simulink model "vision_processing"  (Simulink 7.7)
settings: Solver=FixedStepDiscrete  StartTime=0.0  StopTime=inf  FixedStep=0.05  RelTol=1e-3
undefined symbols (not defined in the file): darwinop_communication_setup
libraries: simulink x16, lib_darwinop x1
settings Model: Creator=florent  LastModifiedBy=eleve
settings DataIOCC: SignalLoggingSaveFormat=Dataset
settings OptimizationCC: ExpressionDepthLimit=128  OptimizeModelRefInitCode=on  LifeSpan=1
settings DebuggingCC: FcnCallInpInsideContextMsg=Enable All
settings HardwareCC: ProdEndianess=LittleEndian  ProdHWDeviceType=Generic->32-bit Embedded Processor
settings RTWCC: SystemTargetFile=darwinoplib.tlc  GenCodeOnly=on  TemplateMakefile=darwinoplib.tmf  Description=DarwinOP code generator  ProcessScript=darwinoplib_make_rtw_hook  TargetLang=C++
settings CodeAppCC: IgnoreCustomStorageClasses=off  CustomSymbolStrType=$N$R$M_T
settings STFCustomTargetCC: CombineOutputUpdateFcns=on  ERTCustomFileBanners=on  SupportContinuousTime=off  SupportNonInlinedSFcns=off  SystemTargetFile=darwinoplib.tlc
settings ERTTargetCC: MultiwordLength=2048  ParMdlRefBuildCompliant=off  CompOptLevelCompliant=off  ERTFirstTimeCompliant=off  ModelStepFunctionPrototypeControlCompliant=off  CPPClassGenCompliant=off  ExtModeMexArgs='192.168.123.1' 1 17725  InlinedParameterPlacement=NonHierarchical  ERTCustomFileTemplate=darwinoplib_main.tlc  ConvertIfToSwitch=off  SuppressUnreachableDefaultCases=off
settings CustomProperty: DataType=string  Value=192.168.123.1

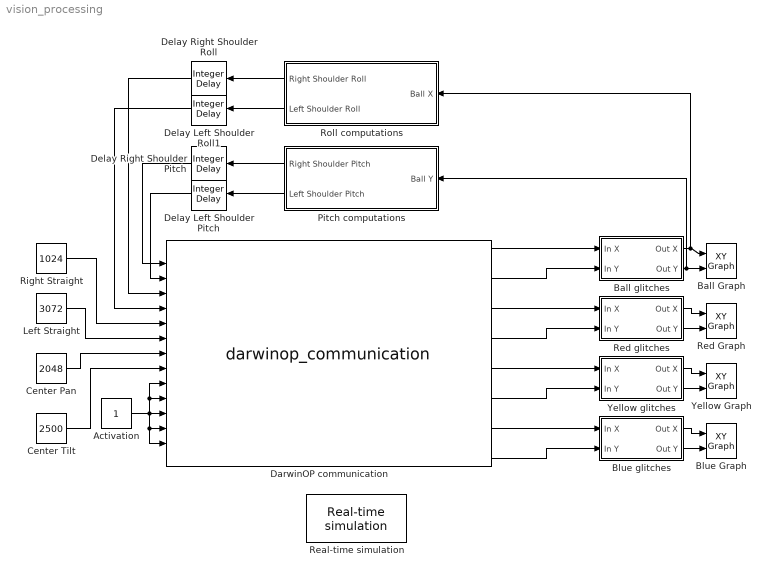
== system vision_processing ==
  Activation : Constant
  Ball Graph : simulink/Sinks/XY Graph  xmin=0  xmax=320  ymin=0  ymax=240  st=-1
  Ball glitches : Subsystem
  Blue Graph : simulink/Sinks/XY Graph  xmin=0  xmax=320  ymin=0  ymax=240  st=-1
  Blue glitches : Subsystem
  Center Pan : Constant  Value=2048
  Center Tilt : Constant  Value=2500
  DarwinOP communication : M-S-Function  StartFcn=darwinop_communication_setup('StartFcn');  StopFcn=darwinop_communication_setup('StopFcn');  FunctionName=darwinop_communication  Parameters=IP,Port,Protocol,Timeout,Frame,ReadIndex,WriteIndex  mask{IP=192.168.123.1, Port=1234, Protocol=tcp, Timeout=0.05, Frame=[ 3 1 30 2 0 0 3 2 30 2 0 0 3 3 30 2 0 0 3 4 30 2 0 0 3 5 30 2 0 0 3 6 30 2 0 0 3 19 30 2 0 0 3 20 30 2 0 0 17 1 30 4 17 1 50 4 17 1 70 4 17 1 90 4 18 1 1 5 0 0 0 0 0], ReadIndex=[ 1 2;3 2;5 2;7 2;9 2;11 2;13 2;15 2], WriteIndex=[ 5 2;11 2;17 2;23 2;29 2;35 2;41 2;47 2;69 1;70 1;71 1;72 1;73 1]}
      settings: DeleteFcn=darwinop_communication_setup('DeleteFcn');  ModelCloseFcn=darwinop_communication_setup('ModelCloseFcn');  NameChangeFcn=darwinop_communication_setup('NameChangeFcn');  OpenFcn=darwinop_communication_setup('OpenFcn');
      mask StyleString: edit,edit,popup(tcp|udp),edit,edit,edit,edit
      mask Display:
      | image(imread('darwin-blk.jpg'))
      | 
      | port_label('output',1,'Vision(1)/Ball X')
      | port_label('output',2,'Vision(1)/Ball Y')
      | port_label('output',3,'Vision(1)/Red X')
      | port_label('output',4,'Vision(1)/Red Y')
      | port_label('output',5,'Vision(1)/Yellow X')
      | port_label('output',6,'Vision(1)/Yellow Y')
      | port_label('output',7,'Vision(1)/Blue X')
      | port_label('output',8,'Vision(1)/Blue Y')
      | 
      | port_label('input',1,'Right Shoulder Pitch(1)/Goal Position')
      | port_label('input',2,'Left Shoulder Pitch(2)/Goal Position')
      | port_label('input',3,'Right Shoulder Roll(3)/Goal Position')
      | port_label('input',4,'Left Shoulder Roll(4)/Goal Position')
      | port_label('input',5,'Right Elbow(5)/Goal Position')
      | port_label('input',6,'Left Elbow(6)/Goal Position')
      | port_label('input',7,'Head Pan(19)/Goal Position')
      | port_label('input',8,'Head Tilt(20)/Goal Position')
      | port_label('input',9,'Vision(1)/Enable')
      | port_label('input',10,'Vision(1)/Ball enable')
      | port_label('input',11,'Vision(1)/Red enable')
      | port_label('input',12,'Vision(1)/Yellow enable')
      | port_label('input',13,'Vision(1)/Blue enable')
  Delay Left Shoulder Pitch : simulink/Discrete/Integer Delay  NumDelays=1  vinit=2048  samptime=-1
  Delay Left Shoulder Roll1 : simulink/Discrete/Integer Delay  NumDelays=1  vinit=2048  samptime=-1
  Delay Right Shoulder Pitch : simulink/Discrete/Integer Delay  NumDelays=1  vinit=2048  samptime=-1
  Delay Right Shoulder Roll : simulink/Discrete/Integer Delay  NumDelays=1  vinit=2048  samptime=-1
  Left Straight : Constant  Value=3072
  Pitch computations : Subsystem
  Real-time simulation : lib_darwinop/Real-time simulation  TimeScalingFactor=1
  Red Graph : simulink/Sinks/XY Graph  xmin=0  xmax=320  ymin=0  ymax=240  st=-1
  Red glitches : Subsystem
  Right Straight : Constant  Value=1024
  Roll computations : Subsystem
  Yellow Graph : simulink/Sinks/XY Graph  xmin=0  xmax=320  ymin=0  ymax=240  st=-1
  Yellow glitches : Subsystem
  wires:
  DarwinOP communication/1 -> Ball glitches/1(In X)
  Ball glitches/1(Out X) -> Roll computations/1(Ball X), Ball Graph/1
  DarwinOP communication/2 -> Ball glitches/2(In Y)
  Ball glitches/2(Out Y) -> Pitch computations/1(Ball Y), Ball Graph/2
  DarwinOP communication/3 -> Red glitches/1(In X)
  Red glitches/1(Out X) -> Red Graph/1
  DarwinOP communication/4 -> Red glitches/2(In Y)
  Red glitches/2(Out Y) -> Red Graph/2
  DarwinOP communication/5 -> Yellow glitches/1(In X)
  Yellow glitches/1(Out X) -> Yellow Graph/1
  DarwinOP communication/6 -> Yellow glitches/2(In Y)
  Yellow glitches/2(Out Y) -> Yellow Graph/2
  DarwinOP communication/7 -> Blue glitches/1(In X)
  Blue glitches/1(Out X) -> Blue Graph/1
  DarwinOP communication/8 -> Blue glitches/2(In Y)
  Blue glitches/2(Out Y) -> Blue Graph/2
  Activation/1 -> DarwinOP communication/10, DarwinOP communication/9, DarwinOP communication/11, DarwinOP communication/12, DarwinOP communication/13
  Center Pan/1 -> DarwinOP communication/7
  Right Straight/1 -> DarwinOP communication/5
  Left Straight/1 -> DarwinOP communication/6
  Pitch computations/1(Right Shoulder Pitch) -> Delay Right Shoulder Pitch/1
  Pitch computations/2(Left Shoulder Pitch) -> Delay Left Shoulder Pitch/1
  Roll computations/1(Right Shoulder Roll) -> Delay Right Shoulder Roll/1
  Roll computations/2(Left Shoulder Roll) -> Delay Left Shoulder Roll1/1
  Center Tilt/1 -> DarwinOP communication/8
  Delay Right Shoulder Roll/1 -> DarwinOP communication/3
  Delay Left Shoulder Roll1/1 -> DarwinOP communication/4
  Delay Right Shoulder Pitch/1 -> DarwinOP communication/1
  Delay Left Shoulder Pitch/1 -> DarwinOP communication/2

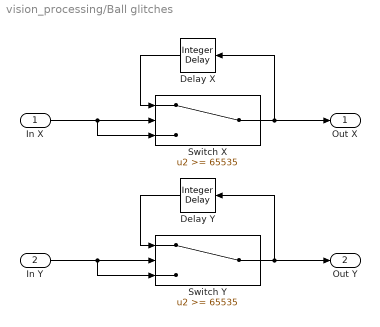
== system vision_processing/Ball glitches ==
  In X : Inport
  In Y : Inport  Port=2
  Delay X : simulink/Discrete/Integer Delay  NumDelays=1  vinit=0.0  samptime=-1
  Delay Y : simulink/Discrete/Integer Delay  NumDelays=1  vinit=0.0  samptime=-1
  Switch X : Switch  Threshold=65535
  Switch Y : Switch  Threshold=65535
  Out X : Outport
  Out Y : Outport  Port=2
  wires:
  Delay X/1 -> Switch X/1
  Switch X/1 -> Out X/1, Delay X/1
  In X/1 -> Switch X/3, Switch X/2
  Delay Y/1 -> Switch Y/1
  Switch Y/1 -> Out Y/1, Delay Y/1
  In Y/1 -> Switch Y/3, Switch Y/2

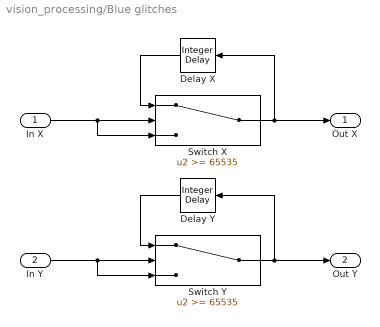
== system vision_processing/Blue glitches ==
  In X : Inport
  In Y : Inport  Port=2
  Delay X : simulink/Discrete/Integer Delay  NumDelays=1  vinit=0.0  samptime=-1
  Delay Y : simulink/Discrete/Integer Delay  NumDelays=1  vinit=0.0  samptime=-1
  Switch X : Switch  Threshold=65535
  Switch Y : Switch  Threshold=65535
  Out X : Outport
  Out Y : Outport  Port=2
  wires:
  Delay X/1 -> Switch X/1
  Switch X/1 -> Out X/1, Delay X/1
  In X/1 -> Switch X/3, Switch X/2
  Delay Y/1 -> Switch Y/1
  Switch Y/1 -> Out Y/1, Delay Y/1
  In Y/1 -> Switch Y/3, Switch Y/2

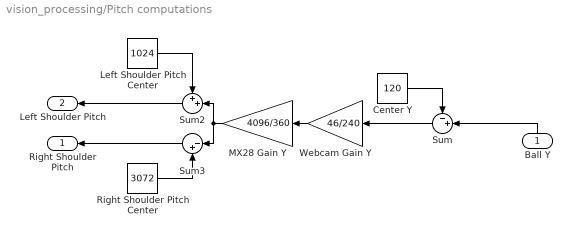
== system vision_processing/Pitch computations ==
  Ball Y : Inport
  Center Y : Constant  Value=120
  Left Shoulder Pitch Center : Constant  Value=1024
  MX28 Gain Y : Gain  Gain=4096/360
  Right Shoulder Pitch Center : Constant  Value=3072
  Sum : Sum  Inputs=-+|
  Sum2 : Sum  Inputs=++|
  Sum3 : Sum  Inputs=|-+
  Webcam Gain Y : Gain  Gain=46/240
  Right Shoulder Pitch : Outport
  Left Shoulder Pitch : Outport  Port=2
  wires:
  Sum/1 -> Webcam Gain Y/1
  Webcam Gain Y/1 -> MX28 Gain Y/1
  Center Y/1 -> Sum/1
  Right Shoulder Pitch Center/1 -> Sum3/2
  Sum3/1 -> Right Shoulder Pitch/1
  Left Shoulder Pitch Center/1 -> Sum2/1
  MX28 Gain Y/1 -> Sum3/1, Sum2/2
  Sum2/1 -> Left Shoulder Pitch/1
  Ball Y/1 -> Sum/2

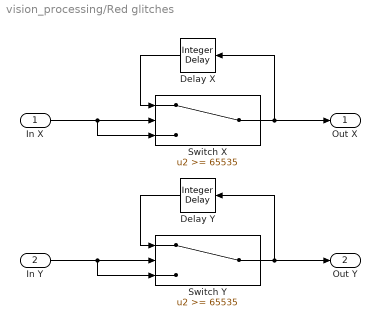
== system vision_processing/Red glitches ==
  In X : Inport
  In Y : Inport  Port=2
  Delay X : simulink/Discrete/Integer Delay  NumDelays=1  vinit=0.0  samptime=-1
  Delay Y : simulink/Discrete/Integer Delay  NumDelays=1  vinit=0.0  samptime=-1
  Switch X : Switch  Threshold=65535
  Switch Y : Switch  Threshold=65535
  Out X : Outport
  Out Y : Outport  Port=2
  wires:
  Delay X/1 -> Switch X/1
  Switch X/1 -> Out X/1, Delay X/1
  In X/1 -> Switch X/3, Switch X/2
  Delay Y/1 -> Switch Y/1
  Switch Y/1 -> Out Y/1, Delay Y/1
  In Y/1 -> Switch Y/3, Switch Y/2

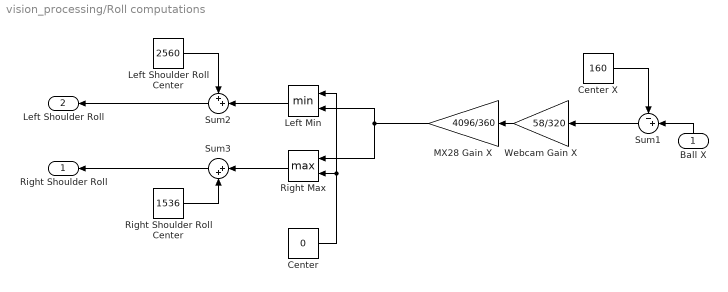
== system vision_processing/Roll computations ==
  Ball X : Inport
  Center : Constant  Value=0
  Center X : Constant  Value=160
  Left Min : MinMax  Inputs=2
  Left Shoulder Roll Center : Constant  Value=2560
  MX28 Gain X : Gain  Gain=4096/360
  Right Max : MinMax  Function=max  Inputs=2
  Right Shoulder Roll Center : Constant  Value=1536
  Sum1 : Sum  Inputs=-+|
  Sum2 : Sum  Inputs=++|
  Sum3 : Sum  Inputs=|++
  Webcam Gain X : Gain  Gain=58/320
  Right Shoulder Roll : Outport
  Left Shoulder Roll : Outport  Port=2
  wires:
  Sum1/1 -> Webcam Gain X/1
  Webcam Gain X/1 -> MX28 Gain X/1
  Center X/1 -> Sum1/1
  Sum2/1 -> Left Shoulder Roll/1
  Sum3/1 -> Right Shoulder Roll/1
  Left Shoulder Roll Center/1 -> Sum2/1
  Right Shoulder Roll Center/1 -> Sum3/2
  Ball X/1 -> Sum1/2
  Left Min/1 -> Sum2/2
  MX28 Gain X/1 -> Left Min/2, Right Max/1
  Right Max/1 -> Sum3/1
  Center/1 -> Right Max/2, Left Min/1

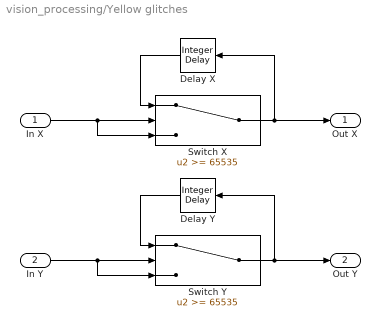
== system vision_processing/Yellow glitches ==
  In X : Inport
  In Y : Inport  Port=2
  Delay X : simulink/Discrete/Integer Delay  NumDelays=1  vinit=0.0  samptime=-1
  Delay Y : simulink/Discrete/Integer Delay  NumDelays=1  vinit=0.0  samptime=-1
  Switch X : Switch  Threshold=65535
  Switch Y : Switch  Threshold=65535
  Out X : Outport
  Out Y : Outport  Port=2
  wires:
  Delay X/1 -> Switch X/1
  Switch X/1 -> Out X/1, Delay X/1
  In X/1 -> Switch X/3, Switch X/2
  Delay Y/1 -> Switch Y/1
  Switch Y/1 -> Out Y/1, Delay Y/1
  In Y/1 -> Switch Y/3, Switch Y/2
